simulink model "Semi_Active_Quarter_Model"  (R2016a)
settings: Solver=ode4  StartTime=0.0  StopTime=Tend  FixedStep=Ts  RelTol=1e-3
values from neighbouring files (symbols this model uses):
  A = [      0      1      0     -1 ... (first row only)    [Semi_Active_Optical_Control.m]
  An = [      0      1      0     -1 ... (first row only)    [Semi_Active_Optical_Control.m]
  B0 = [0 1/m2 0 -1/m1]'    [Semi_Active_Optical_Control.m]
  C = [eye(4);A(2,:); 1 0 1 0]    [Semi_Active_Optical_Control.m]
  c2 = 1000    [Semi_Active_Optical_Control.m]
  Cmax = 3000    [Semi_Active_Optical_Control.m]
  D = [0 0 0 0 B0(2) 0]'    [Semi_Active_Optical_Control.m]
  E = [0 0 0 0 0 1]'    [Semi_Active_Optical_Control.m]
  fr = 1    [Semi_Active_Optical_Control.m]
  k2 = 16000    [Semi_Active_Optical_Control.m]
  m2 = 240    [Semi_Active_Optical_Control.m]
  R0 = 1/(m2)^2    (= 1.73611111111e-05)    [Semi_Active_Optical_Control.m]
  S0 = [-k2/(m2)^2 -c2/(m2)^2 0 c2/(m2)^2]    [Semi_Active_Optical_Control.m]
  SW = 1    [Semi_Active_Optical_Control.m]
  Ts = 0.001    [Semi_Active_Optical_Control.m]
  W = [0 0 -1 0]'    [Semi_Active_Optical_Control.m]
undefined symbols (not defined in the file or in its folder): P
settings Model: Creator=DONLAP140203  LastModifiedBy=DONLAP140203

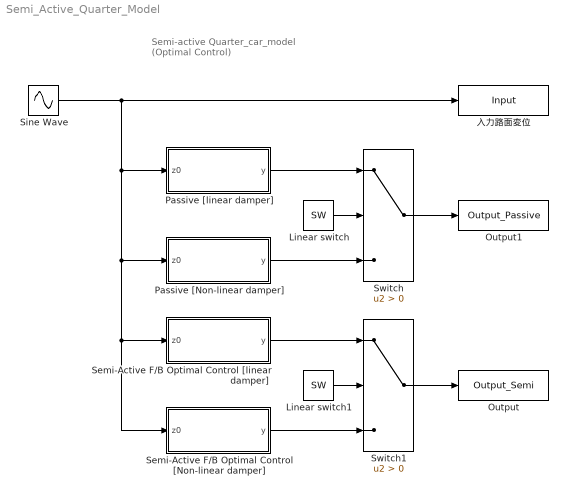
== system Semi_Active_Quarter_Model ==
  note: Semi-active
      | Quarter_car_model
      | (Optimal Control)
  Linear switch : Constant  Value=SW
  Linear switch1 : Constant  Value=SW
  Output : ToWorkspace  VariableName=Output_Semi  SampleTime=-1
  Output1 : ToWorkspace  VariableName=Output_Passive  SampleTime=-1
  Passive [Non-linear damper] : Subsystem
  Passive [linear damper] : Subsystem
  Semi-Active F/B Optimal Control [Non-linear damper] : Subsystem
  Semi-Active F/B Optimal Control [linear damper] : Subsystem
  Sine Wave : Sin  Amplitude=0.05  Frequency=2*pi*fr  SampleTime=0
  Switch : Switch  Criteria=u2 > Threshold
  Switch1 : Switch  Criteria=u2 > Threshold
  入力路面変位 : ToWorkspace  VariableName=Input  SampleTime=-1
  wires:
  Sine Wave/1 -> Semi-Active F/B Optimal Control [Non-linear damper]/1(z0), Semi-Active F/B Optimal Control [linear damper]/1(z0), Passive [Non-linear damper]/1(z0), Passive [linear damper]/1(z0), 入力路面変位/1
  Switch/1 -> Output1/1
  Passive [linear damper]/1(y) -> Switch/1
  Passive [Non-linear damper]/1(y) -> Switch/3
  Linear switch/1 -> Switch/2
  Semi-Active F/B Optimal Control [Non-linear damper]/1(y) -> Switch1/3
  Semi-Active F/B Optimal Control [linear damper]/1(y) -> Switch1/1
  Switch1/1 -> Output/1
  Linear switch1/1 -> Switch1/2

== system Semi_Active_Quarter_Model/Passive [Non-linear damper] ==
  z0 : Inport
  Vehicle 1/4 Model [Non-linear damper] : Subsystem
  control force : Constant  Value=0
  y : Outport
  wires:
  z0/1 -> Vehicle 1/4 Model [Non-linear damper]/1(z0)
  Vehicle 1/4 Model [Non-linear damper]/1(y) -> y/1
  control force/1 -> Vehicle 1/4 Model [Non-linear damper]/2(fc)

== system Semi_Active_Quarter_Model/Passive [linear damper] ==
  z0 : Inport
  Vehicle 1/4 Model [linear damper] : Subsystem
  control force : Constant  Value=0
  y : Outport
  wires:
  z0/1 -> Vehicle 1/4 Model [linear damper]/1(z0)
  Vehicle 1/4 Model [linear damper]/1(y) -> y/1
  control force/1 -> Vehicle 1/4 Model [linear damper]/2(fc)

== system Semi_Active_Quarter_Model/Semi-Active F//B Optimal Control [Non-linear damper] ==
  z0 : Inport
  F/B Optimal Controller [Non-linear damper] : Subsystem
  Vehicle 1/4 Model [Non-linear damper] : Subsystem
  y : Outport
  wires:
  z0/1 -> Vehicle 1/4 Model [Non-linear damper]/1(z0)
  Vehicle 1/4 Model [Non-linear damper]/1(y) -> y/1
  Vehicle 1/4 Model [Non-linear damper]/2(x) -> F/B Optimal Controller [Non-linear damper]/1(x)
  F/B Optimal Controller [Non-linear damper]/1(fc) -> Vehicle 1/4 Model [Non-linear damper]/2(fc)

== system Semi_Active_Quarter_Model/Semi-Active F//B Optimal Control [linear damper] ==
  z0 : Inport
  F/B Optimal Controller : Subsystem
  Vehicle 1/4 Model [linear damper] : Subsystem
  y : Outport
  wires:
  z0/1 -> Vehicle 1/4 Model [linear damper]/1(z0)
  Vehicle 1/4 Model [linear damper]/1(y) -> y/1
  Vehicle 1/4 Model [linear damper]/2(x) -> F/B Optimal Controller/1(x)
  F/B Optimal Controller/1(fc) -> Vehicle 1/4 Model [linear damper]/2(fc)

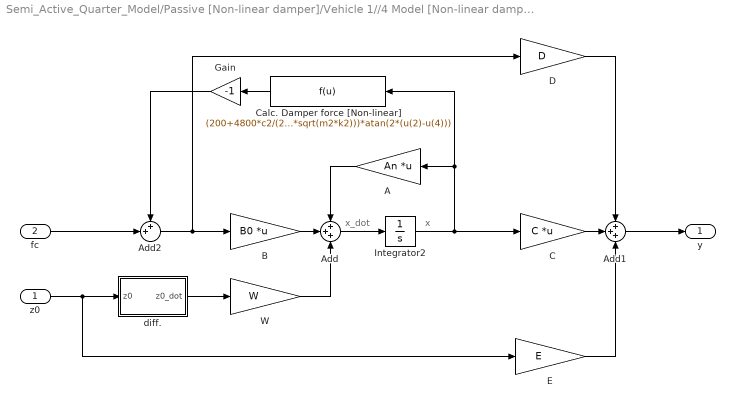
== system Semi_Active_Quarter_Model/Passive [Non-linear damper]/Vehicle 1//4 Model [Non-linear damper] ==
  note: x
  note: x_dot
  z0 : Inport
  fc : Inport  Port=2
  A : Gain  Gain=An  Multiplication=Matrix(K*u) (u vector)
  Add : Sum  Inputs=+++
  Add1 : Sum  Inputs=+++
  Add2 : Sum  Inputs=++|
  B : Gain  Gain=B0  Multiplication=Matrix(K*u) (u vector)
  C : Gain  Gain=C  Multiplication=Matrix(K*u) (u vector)
  Calc. Damper force [Non-linear] : Fcn  Expr=(200+4800*c2/(2*sqrt(m2*k2)))*atan(2*(u(2)-u(4)))
  D : Gain  Gain=D
  E : Gain  Gain=E
  Gain : Gain  Gain=-1
  Integrator2 : Integrator
  W : Gain  Gain=W
  diff. : Subsystem
  y : Outport
  wires:
  Add/1 -> Integrator2/1
  Integrator2/1 -> Calc. Damper force [Non-linear]/1, A/1, C/1
  D/1 -> Add1/1
  C/1 -> Add1/2
  A/1 -> Add/1
  W/1 -> Add/3
  B/1 -> Add/2
  z0/1 -> E/1, diff./1(z0)
  Add1/1 -> y/1
  diff./1(z0_dot) -> W/1
  E/1 -> Add1/3
  Add2/1 -> D/1, B/1
  fc/1 -> Add2/2
  Calc. Damper force [Non-linear]/1 -> Gain/1
  Gain/1 -> Add2/1

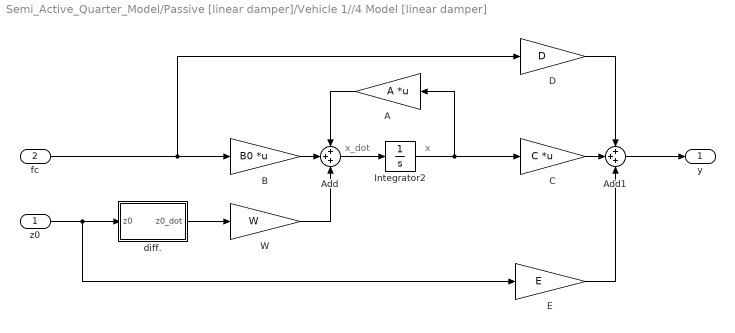
== system Semi_Active_Quarter_Model/Passive [linear damper]/Vehicle 1//4 Model [linear damper] ==
  note: x
  note: x_dot
  z0 : Inport
  fc : Inport  Port=2
  A : Gain  Gain=A  Multiplication=Matrix(K*u) (u vector)
  Add : Sum  Inputs=+++
  Add1 : Sum  Inputs=+++
  B : Gain  Gain=B0  Multiplication=Matrix(K*u) (u vector)
  C : Gain  Gain=C  Multiplication=Matrix(K*u) (u vector)
  D : Gain  Gain=D
  E : Gain  Gain=E
  Integrator2 : Integrator
  W : Gain  Gain=W
  diff. : Subsystem
  y : Outport
  wires:
  Add/1 -> Integrator2/1
  Integrator2/1 -> A/1, C/1
  D/1 -> Add1/1
  C/1 -> Add1/2
  fc/1 -> D/1, B/1
  A/1 -> Add/1
  W/1 -> Add/3
  B/1 -> Add/2
  z0/1 -> E/1, diff./1(z0)
  Add1/1 -> y/1
  diff./1(z0_dot) -> W/1
  E/1 -> Add1/3

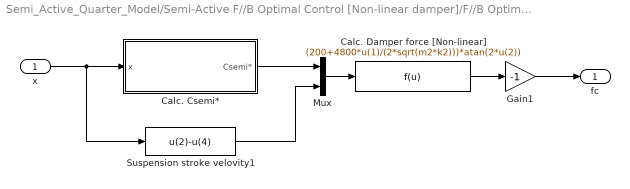
== system Semi_Active_Quarter_Model/Semi-Active F//B Optimal Control [Non-linear damper]/F//B Optimal Controller [Non-linear damper] ==
  x : Inport
  Calc. Csemi* : Subsystem
  Calc. Damper force [Non-linear] : Fcn  Expr=(200+4800*u(1)/(2*sqrt(m2*k2)))*atan(2*u(2))
  Gain1 : Gain  Gain=-1
  Mux : Mux  Inputs=2
  Suspension stroke velovity1 : Fcn  Expr=u(2)-u(4)
  fc : Outport
  wires:
  x/1 -> Suspension stroke velovity1/1, Calc. Csemi*/1(x)
  Suspension stroke velovity1/1 -> Mux/2
  Mux/1 -> Calc. Damper force [Non-linear]/1
  Calc. Damper force [Non-linear]/1 -> Gain1/1
  Gain1/1 -> fc/1
  Calc. Csemi*/1(Csemi*) -> Mux/1

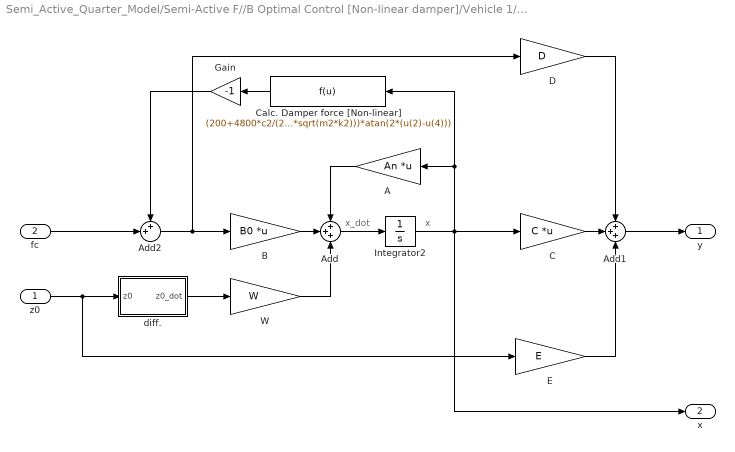
== system Semi_Active_Quarter_Model/Semi-Active F//B Optimal Control [Non-linear damper]/Vehicle 1//4 Model [Non-linear damper] ==
  note: x
  note: x_dot
  z0 : Inport
  fc : Inport  Port=2
  A : Gain  Gain=An  Multiplication=Matrix(K*u) (u vector)
  Add : Sum  Inputs=+++
  Add1 : Sum  Inputs=+++
  Add2 : Sum  Inputs=++|
  B : Gain  Gain=B0  Multiplication=Matrix(K*u) (u vector)
  C : Gain  Gain=C  Multiplication=Matrix(K*u) (u vector)
  Calc. Damper force [Non-linear] : Fcn  Expr=(200+4800*c2/(2*sqrt(m2*k2)))*atan(2*(u(2)-u(4)))
  D : Gain  Gain=D
  E : Gain  Gain=E
  Gain : Gain  Gain=-1
  Integrator2 : Integrator
  W : Gain  Gain=W
  diff. : Subsystem
  y : Outport
  x : Outport  Port=2
  wires:
  Add/1 -> Integrator2/1
  Integrator2/1 -> Calc. Damper force [Non-linear]/1, A/1, x/1, C/1
  D/1 -> Add1/1
  C/1 -> Add1/2
  A/1 -> Add/1
  W/1 -> Add/3
  B/1 -> Add/2
  z0/1 -> E/1, diff./1(z0)
  Add1/1 -> y/1
  diff./1(z0_dot) -> W/1
  E/1 -> Add1/3
  Add2/1 -> D/1, B/1
  fc/1 -> Add2/2
  Calc. Damper force [Non-linear]/1 -> Gain/1
  Gain/1 -> Add2/1

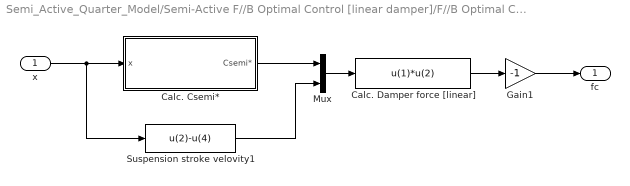
== system Semi_Active_Quarter_Model/Semi-Active F//B Optimal Control [linear damper]/F//B Optimal Controller ==
  x : Inport
  Calc. Csemi* : Subsystem
  Calc. Damper force [linear] : Fcn  Expr=u(1)*u(2)
  Gain1 : Gain  Gain=-1
  Mux : Mux  Inputs=2
  Suspension stroke velovity1 : Fcn  Expr=u(2)-u(4)
  fc : Outport
  wires:
  x/1 -> Suspension stroke velovity1/1, Calc. Csemi*/1(x)
  Suspension stroke velovity1/1 -> Mux/2
  Mux/1 -> Calc. Damper force [linear]/1
  Calc. Damper force [linear]/1 -> Gain1/1
  Gain1/1 -> fc/1
  Calc. Csemi*/1(Csemi*) -> Mux/1

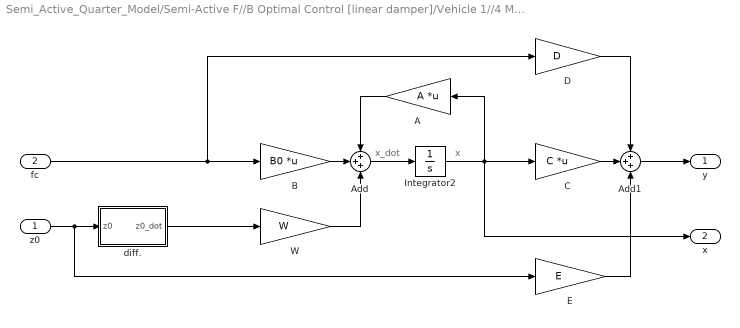
== system Semi_Active_Quarter_Model/Semi-Active F//B Optimal Control [linear damper]/Vehicle 1//4 Model [linear damper] ==
  note: x
  note: x_dot
  z0 : Inport
  fc : Inport  Port=2
  A : Gain  Gain=A  Multiplication=Matrix(K*u) (u vector)
  Add : Sum  Inputs=+++
  Add1 : Sum  Inputs=+++
  B : Gain  Gain=B0  Multiplication=Matrix(K*u) (u vector)
  C : Gain  Gain=C  Multiplication=Matrix(K*u) (u vector)
  D : Gain  Gain=D
  E : Gain  Gain=E
  Integrator2 : Integrator
  W : Gain  Gain=W
  diff. : Subsystem
  y : Outport
  x : Outport  Port=2
  wires:
  Add/1 -> Integrator2/1
  Integrator2/1 -> A/1, x/1, C/1
  D/1 -> Add1/1
  C/1 -> Add1/2
  fc/1 -> D/1, B/1
  A/1 -> Add/1
  W/1 -> Add/3
  B/1 -> Add/2
  z0/1 -> E/1, diff./1(z0)
  Add1/1 -> y/1
  diff./1(z0_dot) -> W/1
  E/1 -> Add1/3

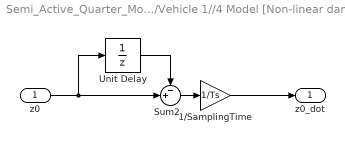
== system Semi_Active_Quarter_Model/Passive [Non-linear damper]/Vehicle 1//4 Model [Non-linear damper]/diff. ==
  z0 : Inport
  1/SamplingTime : Gain  Gain=1/Ts
  Sum2 : Sum  Inputs=-+|
  Unit Delay : UnitDelay  SampleTime=-1
  z0_dot : Outport
  wires:
  Sum2/1 -> 1/SamplingTime/1
  1/SamplingTime/1 -> z0_dot/1
  Unit Delay/1 -> Sum2/1
  z0/1 -> Sum2/2, Unit Delay/1

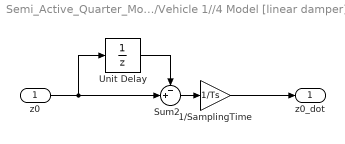
== system Semi_Active_Quarter_Model/Passive [linear damper]/Vehicle 1//4 Model [linear damper]/diff. ==
  z0 : Inport
  1/SamplingTime : Gain  Gain=1/Ts
  Sum2 : Sum  Inputs=-+|
  Unit Delay : UnitDelay  SampleTime=-1
  z0_dot : Outport
  wires:
  Sum2/1 -> 1/SamplingTime/1
  1/SamplingTime/1 -> z0_dot/1
  Unit Delay/1 -> Sum2/1
  z0/1 -> Sum2/2, Unit Delay/1

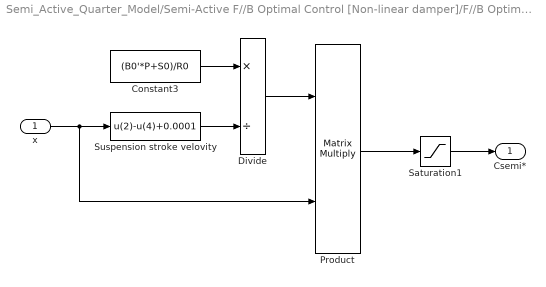
== system Semi_Active_Quarter_Model/Semi-Active F//B Optimal Control [Non-linear damper]/F//B Optimal Controller [Non-linear damper]/Calc. Csemi* ==
  x : Inport
  Constant3 : Constant  Value=(B0'*P+S0)/R0  VectorParams1D=off
  Divide : Product  Inputs=*/
  Product : Product  Multiplication=Matrix(*)
  Saturation1 : Saturate  UpperLimit=Cmax  LowerLimit=0
  Suspension stroke velovity : Fcn  Expr=u(2)-u(4)+0.0001
  Csemi* : Outport
  wires:
  Product/1 -> Saturation1/1
  Saturation1/1 -> Csemi*/1
  Constant3/1 -> Divide/1
  Suspension stroke velovity/1 -> Divide/2
  Divide/1 -> Product/1
  x/1 -> Product/2, Suspension stroke velovity/1

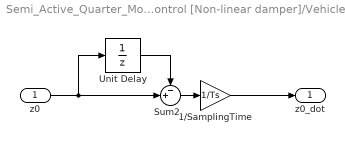
== system Semi_Active_Quarter_Model/Semi-Active F//B Optimal Control [Non-linear damper]/Vehicle 1//4 Model [Non-linear damper]/diff. ==
  z0 : Inport
  1/SamplingTime : Gain  Gain=1/Ts
  Sum2 : Sum  Inputs=-+|
  Unit Delay : UnitDelay  SampleTime=-1
  z0_dot : Outport
  wires:
  Sum2/1 -> 1/SamplingTime/1
  1/SamplingTime/1 -> z0_dot/1
  Unit Delay/1 -> Sum2/1
  z0/1 -> Sum2/2, Unit Delay/1

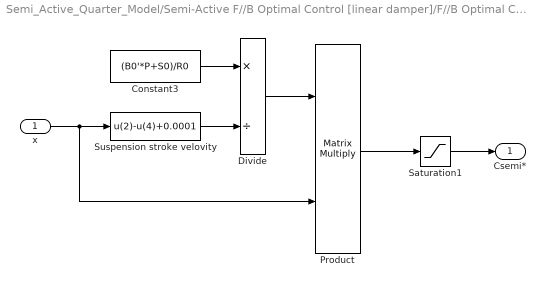
== system Semi_Active_Quarter_Model/Semi-Active F//B Optimal Control [linear damper]/F//B Optimal Controller/Calc. Csemi* ==
  x : Inport
  Constant3 : Constant  Value=(B0'*P+S0)/R0  VectorParams1D=off
  Divide : Product  Inputs=*/
  Product : Product  Multiplication=Matrix(*)
  Saturation1 : Saturate  UpperLimit=Cmax  LowerLimit=0
  Suspension stroke velovity : Fcn  Expr=u(2)-u(4)+0.0001
  Csemi* : Outport
  wires:
  Product/1 -> Saturation1/1
  Saturation1/1 -> Csemi*/1
  Constant3/1 -> Divide/1
  Suspension stroke velovity/1 -> Divide/2
  Divide/1 -> Product/1
  x/1 -> Product/2, Suspension stroke velovity/1

== system Semi_Active_Quarter_Model/Semi-Active F//B Optimal Control [linear damper]/Vehicle 1//4 Model [linear damper]/diff. ==
  z0 : Inport
  1/SamplingTime : Gain  Gain=1/Ts
  Sum2 : Sum  Inputs=-+|
  Unit Delay : UnitDelay  SampleTime=-1
  z0_dot : Outport
  wires:
  Sum2/1 -> 1/SamplingTime/1
  1/SamplingTime/1 -> z0_dot/1
  Unit Delay/1 -> Sum2/1
  z0/1 -> Sum2/2, Unit Delay/1
